simulink model "selmotor4"  (Simulink 2.09)
settings: Solver=VariableStepDiscrete  StartTime=0.0  StopTime=1  FixedStep=0.1  MaxStep=0.01  RelTol=1e-3  AbsTol=1e-6
settings Model: OutputTimes=[1]  SaveTime=off  SaveOutput=off  ConsistencyChecking=off  RTWTemplateMakefile=grt_vc.tmf

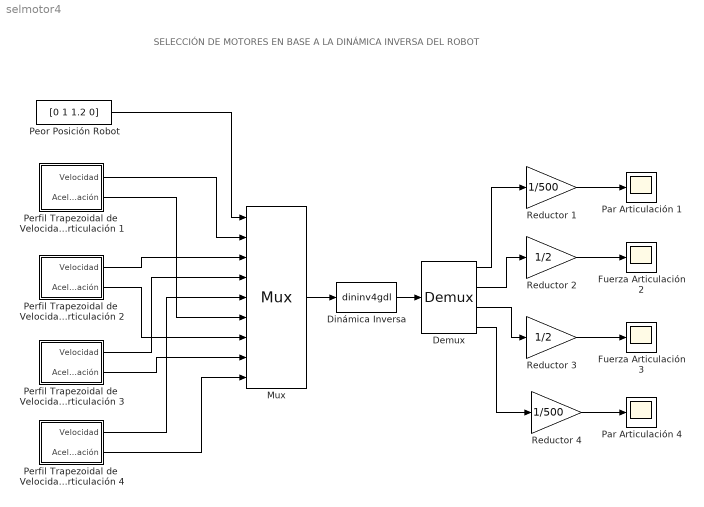
== system selmotor4 ==
  note: SELECCIÓN DE MOTORES EN BASE
      | A LA DINÁMICA INVERSA DEL ROBOT
  Demux : Demux  Outputs=4
  Dinámica Inversa : MATLABFcn  MATLABFcn=dininv4gdl  OutputWidth=4
  Fuerza Articulación 2 : Scope
      settings: TickLabels=on  TimeRange=auto  YMin=-5  YMax=5  SaveToWorkspace=off  SaveName=ScopeData  LimitMaxRows=off
  Fuerza Articulación 3 : Scope
      settings: TickLabels=on  TimeRange=auto  YMin=-5  YMax=5  SaveToWorkspace=off  SaveName=ScopeData  LimitMaxRows=off
  Mux : Mux  Inputs=9
  Par Articulación 1 : Scope
      settings: TickLabels=on  TimeRange=auto  YMin=-0.075  YMax=0.005  SaveToWorkspace=off  SaveName=ScopeData  LimitMaxRows=off
  Par Articulación 4 : Scope
      settings: TickLabels=on  TimeRange=auto  YMin=-5  YMax=5  SaveToWorkspace=off  SaveName=ScopeData  LimitMaxRows=off
  Peor Posición Robot : Constant  Value=[0 1 1.2 0]
  Perfil Trapezoidal de  Velocidad Articulación 1 : Subsystem  mask(Perfil Trapezoidal de Velocidad){velmax=pi/3, tacel=0.1, tconst=0.4, tdecel=0.1}
      mask prompts: velmax "Velocidad máxima"; tacel "Tiempo aceleración"; tconst "Tiempo constante"; tdecel "Tiempo deceleración"
  Perfil Trapezoidal de  Velocidad Articulación 2 : Subsystem  mask(Perfil Trapezoidal de Velocidad){velmax=1, tacel=0.1, tconst=0.4, tdecel=0.1}
      mask prompts: velmax "Velocidad máxima"; tacel "Tiempo aceleración"; tconst "Tiempo constante"; tdecel "Tiempo deceleración"
  Perfil Trapezoidal de  Velocidad Articulación 3 : Subsystem  mask(Perfil Trapezoidal de Velocidad){velmax=1, tacel=0.1, tconst=0.4, tdecel=0.1}
      mask prompts: velmax "Velocidad máxima"; tacel "Tiempo aceleración"; tconst "Tiempo constante"; tdecel "Tiempo deceleración"
  Perfil Trapezoidal de  Velocidad Articulación 4 : Subsystem  mask(Perfil Trapezoidal de Velocidad){velmax=pi/3, tacel=0.1, tconst=0.4, tdecel=0.1}
      mask prompts: velmax "Velocidad máxima"; tacel "Tiempo aceleración"; tconst "Tiempo constante"; tdecel "Tiempo deceleración"
  Reductor 1 : Gain  Gain=1/500
  Reductor 2 : Gain  Gain=1/2
  Reductor 3 : Gain  Gain=1/2
  Reductor 4 : Gain  Gain=1/500
  wires:
  Perfil Trapezoidal de  Velocidad Articulación 4/1(Velocidad) -> Mux/5
  Perfil Trapezoidal de  Velocidad Articulación 3/1(Velocidad) -> Mux/4
  Perfil Trapezoidal de  Velocidad Articulación 2/1(Velocidad) -> Mux/3
  Perfil Trapezoidal de  Velocidad Articulación 1/1(Velocidad) -> Mux/2
  Mux/1 -> Dinámica Inversa/1
  Peor Posición Robot/1 -> Mux/1
  Dinámica Inversa/1 -> Demux/1
  Perfil Trapezoidal de  Velocidad Articulación 1/2(Aceleración) -> Mux/6
  Perfil Trapezoidal de  Velocidad Articulación 2/2(Aceleración) -> Mux/7
  Perfil Trapezoidal de  Velocidad Articulación 3/2(Aceleración) -> Mux/8
  Perfil Trapezoidal de  Velocidad Articulación 4/2(Aceleración) -> Mux/9
  Demux/4 -> Reductor 4/1
  Demux/3 -> Reductor 3/1
  Reductor 4/1 -> Par Articulación 4/1
  Reductor 3/1 -> Fuerza Articulación 3/1
  Demux/2 -> Reductor 2/1
  Demux/1 -> Reductor 1/1
  Reductor 2/1 -> Fuerza Articulación 2/1
  Reductor 1/1 -> Par Articulación 1/1

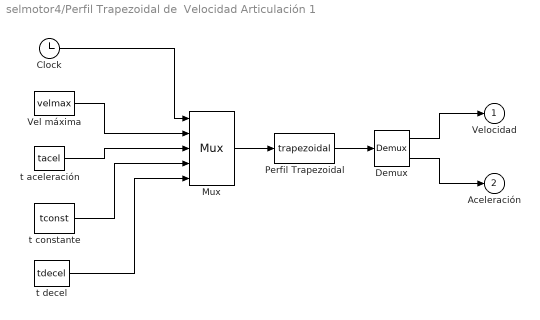
== system selmotor4/Perfil Trapezoidal de  Velocidad Articulación 1 ==
  Clock : Clock
  Demux : Demux  Outputs=2
  Mux : Mux  Inputs=5
  Perfil Trapezoidal : MATLABFcn  MATLABFcn=trapezoidal  OutputWidth=2
  Vel máxima : Constant  Value=velmax
  t aceleración : Constant  Value=tacel
  t constante : Constant  Value=tconst
  t decel : Constant  Value=tdecel
  Velocidad : Outport  Port=1  InitialOutput=0
  Aceleración : Outport  Port=2  InitialOutput=0
  wires:
  Perfil Trapezoidal/1 -> Demux/1
  Demux/2 -> Aceleración/1
  Demux/1 -> Velocidad/1
  Clock/1 -> Mux/1
  Vel máxima/1 -> Mux/2
  t aceleración/1 -> Mux/3
  t constante/1 -> Mux/4
  t decel/1 -> Mux/5
  Mux/1 -> Perfil Trapezoidal/1

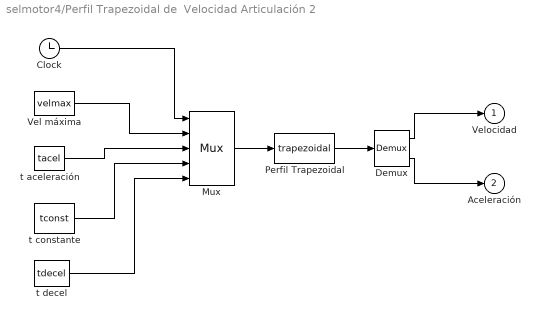
== system selmotor4/Perfil Trapezoidal de  Velocidad Articulación 2 ==
  Clock : Clock
  Demux : Demux  Outputs=2
  Mux : Mux  Inputs=5
  Perfil Trapezoidal : MATLABFcn  MATLABFcn=trapezoidal  OutputWidth=2
  Vel máxima : Constant  Value=velmax
  t aceleración : Constant  Value=tacel
  t constante : Constant  Value=tconst
  t decel : Constant  Value=tdecel
  Velocidad : Outport  Port=1  InitialOutput=0
  Aceleración : Outport  Port=2  InitialOutput=0
  wires:
  Mux/1 -> Perfil Trapezoidal/1
  t decel/1 -> Mux/5
  t constante/1 -> Mux/4
  t aceleración/1 -> Mux/3
  Vel máxima/1 -> Mux/2
  Clock/1 -> Mux/1
  Demux/1 -> Velocidad/1
  Demux/2 -> Aceleración/1
  Perfil Trapezoidal/1 -> Demux/1

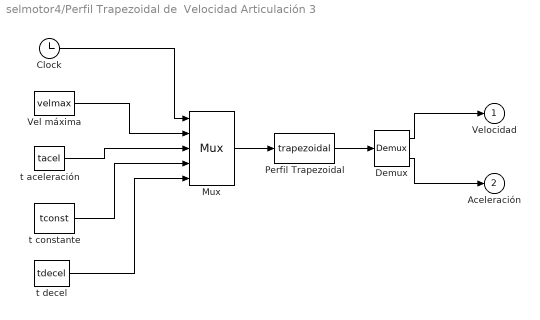
== system selmotor4/Perfil Trapezoidal de  Velocidad Articulación 3 ==
  Clock : Clock
  Demux : Demux  Outputs=2
  Mux : Mux  Inputs=5
  Perfil Trapezoidal : MATLABFcn  MATLABFcn=trapezoidal  OutputWidth=2
  Vel máxima : Constant  Value=velmax
  t aceleración : Constant  Value=tacel
  t constante : Constant  Value=tconst
  t decel : Constant  Value=tdecel
  Velocidad : Outport  Port=1  InitialOutput=0
  Aceleración : Outport  Port=2  InitialOutput=0
  wires:
  Mux/1 -> Perfil Trapezoidal/1
  t decel/1 -> Mux/5
  t constante/1 -> Mux/4
  t aceleración/1 -> Mux/3
  Vel máxima/1 -> Mux/2
  Clock/1 -> Mux/1
  Demux/1 -> Velocidad/1
  Demux/2 -> Aceleración/1
  Perfil Trapezoidal/1 -> Demux/1

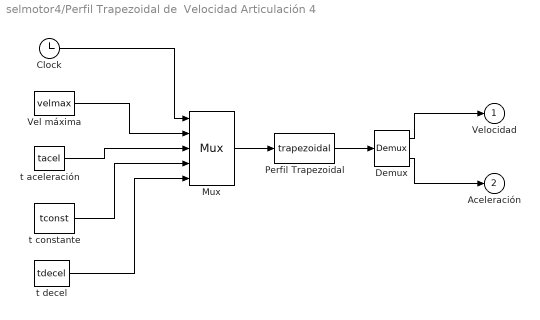
== system selmotor4/Perfil Trapezoidal de  Velocidad Articulación 4 ==
  Clock : Clock
  Demux : Demux  Outputs=2
  Mux : Mux  Inputs=5
  Perfil Trapezoidal : MATLABFcn  MATLABFcn=trapezoidal  OutputWidth=2
  Vel máxima : Constant  Value=velmax
  t aceleración : Constant  Value=tacel
  t constante : Constant  Value=tconst
  t decel : Constant  Value=tdecel
  Velocidad : Outport  Port=1  InitialOutput=0
  Aceleración : Outport  Port=2  InitialOutput=0
  wires:
  Perfil Trapezoidal/1 -> Demux/1
  Demux/2 -> Aceleración/1
  Demux/1 -> Velocidad/1
  Clock/1 -> Mux/1
  Vel máxima/1 -> Mux/2
  t aceleración/1 -> Mux/3
  t constante/1 -> Mux/4
  t decel/1 -> Mux/5
  Mux/1 -> Perfil Trapezoidal/1
